simulink model "LinearBPS_inStateSpace"  (R2023b)
settings: Solver=VariableStepAuto  StartTime=0.0  StopTime=10.0  RelTol=1e-3
settings Model: Creator=msdbg  LastModifiedBy=msdbg

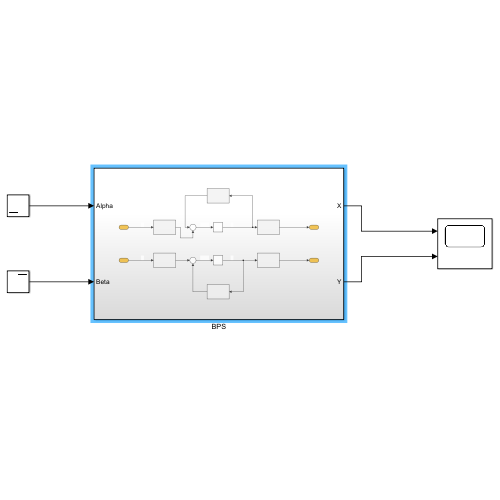
[thumbnail: Simulink's stored preview of the top-level diagram]
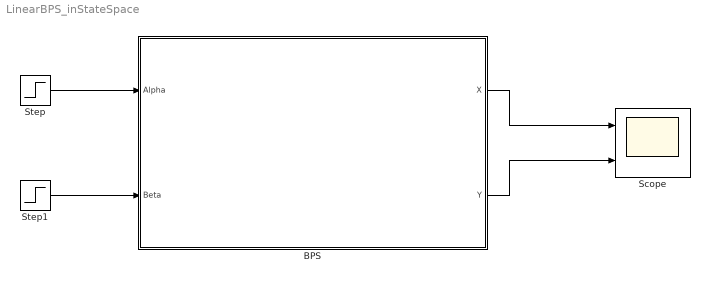
== system LinearBPS_inStateSpace ==
  BPS : Subsystem
  Scope : Scope  NumInputPorts=2
  Step : Step  After=3.14/10  SampleTime=0
  Step1 : Step  After=3.14/10  SampleTime=0
  wires:
  Step/1 -> BPS/1(Alpha)
  BPS/2(Y) -> Scope/2
  Step1/1 -> BPS/2(Beta)
  BPS/1(X) -> Scope/1

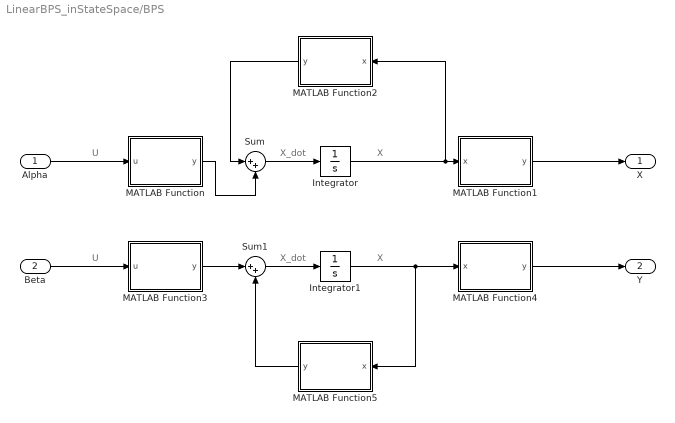
== system LinearBPS_inStateSpace/BPS ==
  note: X
  note: X_dot
  note: U
  note: U
  note: X
  note: X_dot
  Alpha : Inport
  Beta : Inport  Port=2
  Integrator : Integrator
  Integrator1 : Integrator
  MATLAB Function : MATLAB Function  TreatAsAtomicUnit=on
  MATLAB Function1 : MATLAB Function  TreatAsAtomicUnit=on
  MATLAB Function2 : MATLAB Function  TreatAsAtomicUnit=on
  MATLAB Function3 : MATLAB Function  TreatAsAtomicUnit=on
  MATLAB Function4 : MATLAB Function  TreatAsAtomicUnit=on
  MATLAB Function5 : MATLAB Function  TreatAsAtomicUnit=on
  Sum : Sum  Inputs=|++
  Sum1 : Sum  Inputs=|++
  X : Outport
  Y : Outport  Port=2
  wires:
  Alpha/1 -> MATLAB Function/1(u)
  MATLAB Function3/1(y) -> Sum1/1
  Integrator1/1 -> MATLAB Function4/1(x), MATLAB Function5/1(x)
  Beta/1 -> MATLAB Function3/1(u)
  MATLAB Function4/1(y) -> Y/1
  MATLAB Function5/1(y) -> Sum1/2
  Sum/1 -> Integrator/1
  Integrator/1 -> MATLAB Function1/1(x), MATLAB Function2/1(x)
  Sum1/1 -> Integrator1/1
  MATLAB Function1/1(y) -> X/1
  MATLAB Function/1(y) -> Sum/2
  MATLAB Function2/1(y) -> Sum/1

== matlab function LinearBPS_inStateSpace/BPS/MATLAB Function ==
  data: u input; y output
function y = B(u)

y = [0; 5/7*-9.81]*u;

== matlab function LinearBPS_inStateSpace/BPS/MATLAB Function2 ==
  data: x input; y output
function y = A(x)

y = [0 1 ; 0 0]*x;

== matlab function LinearBPS_inStateSpace/BPS/MATLAB Function3 ==
  data: u input; y output
function y = B(u)

y = [0; 5/7*-9.81]*u;

== matlab function LinearBPS_inStateSpace/BPS/MATLAB Function4 ==
  data: x input; y output
function y = C(x)

y = [1 0]*x;

== matlab function LinearBPS_inStateSpace/BPS/MATLAB Function5 ==
  data: x input; y output
function y = A(x)

y = [0 1 ; 0 0]*x;

== matlab function LinearBPS_inStateSpace/BPS/MATLAB Function1 ==
  data: x input; y output
function y = C(x)

y = [1 0]*x;
